simulink library "genset"  (R2014b)
settings: Solver=ode3  StartTime=0.0  StopTime=10.0  RelTol=1e-3
undefined symbols (not defined in the file): AFlowcontrol, AFn, generators, genset, i, Kappa1, ma0, magnitude, nr, pin0, swbId
libraries: goto x6, genset x3, simulink x2, switchboard x1
(part 1 of 2)
settings Model: Creator=torstebo  LastModifiedBy=torstebo

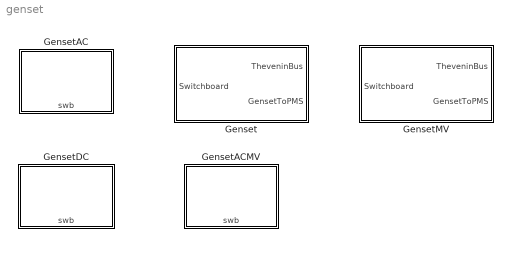
== system genset ==
  Genset : Subsystem
  GensetAC : Subsystem  Tag=GensetAC  mask{genset=generators(1), swbId=1}
      mask prompts: genset "Generator set data"; swbId "SwitchboardId"
      mask Display: image(imread('figs/generator.jpg'),'center')
  GensetACMV : Subsystem  Tag=GensetAC  mask{genset=generators(1), swbId=1}
      mask prompts: genset "Generator set data"; swbId "SwitchboardId"
      mask Display: image(imread('figs/generator.jpg'),'center')
  GensetDC : Subsystem  Tag=GensetDC  mask{genset=generators(1), swbId=1}
      mask prompts: genset "Generator set data"; swbId "SwitchboardId"
      mask Display: image(imread('figs/generator.jpg'),'center')
  GensetMV : Subsystem

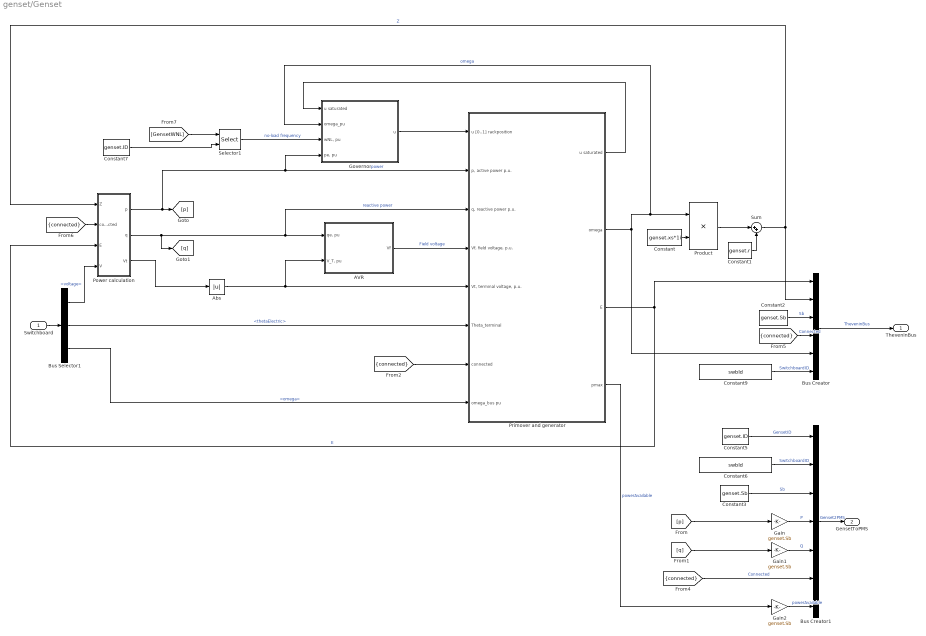
== system genset/Genset ==
  Switchboard : Inport
  AVR : Subsystem
  Abs : Abs
  Bus Creator : BusCreator  Inputs='E','Z','Sb','Connected','omega','SwitchboardID'  OutDataTypeStr=Bus: TheveninBus  NonVirtualBus=on
  Bus Creator1 : BusCreator  Inputs='GensetID','SwitchboardID','Sb','P','Q','Connected','powerAvailable'  OutDataTypeStr=Bus: Genset2PMS  NonVirtualBus=on
  Bus Selector1 : BusSelector  OutputSignals=voltage,thetaElectric,omega
  Constant : Constant  Value=genset.xs*1i
  Constant1 : Constant  Value=genset.r
  Constant2 : Constant  Value=genset.Sb
  Constant3 : Constant  Value=genset.Sb
  Constant5 : Constant  Value=genset.ID  OutDataTypeStr=Inherit: Inherit via back propagation
  Constant6 : Constant  Value=swbId  OutDataTypeStr=Inherit: Inherit via back propagation
  Constant7 : Constant  Value=genset.ID  OutDataTypeStr=Inherit: Inherit via back propagation
  Constant9 : Constant  Value=swbId  OutDataTypeStr=Inherit: Inherit via back propagation
  Gain : Gain  Gain=genset.Sb
  Gain1 : Gain  Gain=genset.Sb
  Gain2 : Gain  Gain=genset.Sb
  Governor : Subsystem
  Power calculation : MATLAB Function  TreatAsAtomicUnit=on
  Primover and generator : Subsystem
  Product : Product
  Selector1 : Selector  IndexOptions=Index vector (port)  Indices=[nr]
  Sum : Sum  Inputs=|++
  TheveninBus : Outport
  GensetToPMS : Outport  Port=2
  wires:
  Bus Selector1/2 -> Primover and generator/6(Theta_terminal)  "<thetaElectric>"
  Constant9/1 -> Bus Creator/6  "SwitchboardID"
  Switchboard/1 -> Bus Selector1/1
  Bus Selector1/3 -> Primover and generator/8(omega_bus pu)  "<omega>"
  Power calculation/3(Vt) -> Abs/1
  [connected] -> Bus Creator/4  "Connected"
  [connected] -> Bus Creator1/6  "Connected"
  [connected] -> Power calculation/2(connected)
  [connected] -> Primover and generator/7(connected)
  Gain2/1 -> Bus Creator1/7  "powerAvailable"
  Bus Selector1/1 -> Power calculation/4(V)  "<voltage>"
  Gain1/1 -> Bus Creator1/5  "Q"
  Gain/1 -> Bus Creator1/4  "P"
  Constant6/1 -> Bus Creator1/2  "SwitchboardID"
  Constant5/1 -> Bus Creator1/1  "GensetID"
  Constant3/1 -> Bus Creator1/3  "Sb"
  Selector1/1 -> Governor/3("wNL, pu")  "no-load frequency"
  AVR/1(Vf) -> Primover and generator/4("Vf, field voltage, p.u.")  "Field voltage"
  Primover and generator/1(u saturated) -> Governor/1(u saturated)
  Primover and generator/2(omega) -> Bus Creator/5, Governor/2(omega_pu), Product/1  "omega"
  Primover and generator/3(E) -> Power calculation/3(E), Bus Creator/1  "E"
  Governor/1(u) -> Primover and generator/1(u [0..1] rackposition)
  [GensetWNL] -> Selector1/1
  Power calculation/1(p) -> Primover and generator/2("p, active power p.u."), Governor/4("pe, pu"), [p]  "power"
  Power calculation/2(q) -> Primover and generator/3("q, reactive power p.u."), AVR/1("qe, pu"), [q]  "reactive power"
  Primover and generator/4(pmax) -> Gain2/1  "powerAvailable"
  Abs/1 -> Primover and generator/5("Vt, terminal voltage, p.u."), AVR/2("V_T, pu")
  Constant/1 -> Product/2
  Product/1 -> Sum/1
  Constant1/1 -> Sum/2
  Sum/1 -> Power calculation/1(Z), Bus Creator/2  "Z"
  Bus Creator/1 -> TheveninBus/1  "TheveninBus"
  Constant2/1 -> Bus Creator/3  "Sb"
  [q] -> Gain1/1
  [p] -> Gain/1
  Constant7/1 -> Selector1/2
  Bus Creator1/1 -> GensetToPMS/1  "Genset2PMS"

== system genset/GensetAC ==
  swb : Inport
  Constant4 : Constant  Value=genset.ID  OutDataTypeStr=Inherit: Inherit via back propagation
  Constant8 : Constant  Value=swbId  OutDataTypeStr=Inherit: Inherit via back propagation
  Genset : genset/Genset
      link override Primover and generator/turbo/Gain2: Gain=genset.turbo.FCdp2
      link override Primover and generator/turbo/Gain4: Gain=genset.turbo.FCdp1
  Goto Tag Visibility : GotoTagVisibility  GotoTag=connected
  Goto3 : goto/Goto  GotoTag=sprintf('Generatorset%d',genset.ID)
  Goto5 : goto/Goto  GotoTag=sprintf('GeneratorsetElectric%d',genset.ID)
  Selector : Selector  IndexOptions=Index vector (port)  Indices=[nr]
  Selector2 : Selector  IndexOptions=Index vector (port)  Indices=[nr]
  Terminator : Terminator
  tag scope: connected=scoped
  wires:
  Constant8/1 -> Selector2/2
  swb/1 -> Terminator/1
  Selector/1 -> [connected]
  [gensetsOn] -> Selector/1  "Connected"
  [switchboard] -> Selector2/1
  Constant4/1 -> Selector/2
  Selector2/1 -> Genset/1
  Genset/1 -> Goto5/1
  Genset/2 -> Goto3/1  "Genset2PMS"

== system genset/GensetACMV ==
  swb : Inport
  Constant4 : Constant  Value=genset.ID  OutDataTypeStr=Inherit: Inherit via back propagation
  Constant8 : Constant  Value=swbId  OutDataTypeStr=Inherit: Inherit via back propagation
  GensetMV : genset/GensetMV
  Goto Tag Visibility : GotoTagVisibility  GotoTag=connected
  Goto3 : goto/Goto  GotoTag=sprintf('Generatorset%d',genset.ID)
  Goto5 : goto/Goto  GotoTag=sprintf('GeneratorsetElectric%d',genset.ID)
  Selector : Selector  IndexOptions=Index vector (port)  Indices=[nr]
  Selector2 : Selector  IndexOptions=Index vector (port)  Indices=[nr]
  Terminator : Terminator
  tag scope: connected=scoped
  wires:
  Constant8/1 -> Selector2/2
  swb/1 -> Terminator/1
  Selector/1 -> [connected]
  [gensetsOn] -> Selector/1  "Connected"
  [switchboard] -> Selector2/1
  Constant4/1 -> Selector/2
  Selector2/1 -> GensetMV/1
  GensetMV/1 -> Goto5/1
  GensetMV/2 -> Goto3/1  "Genset2PMS"

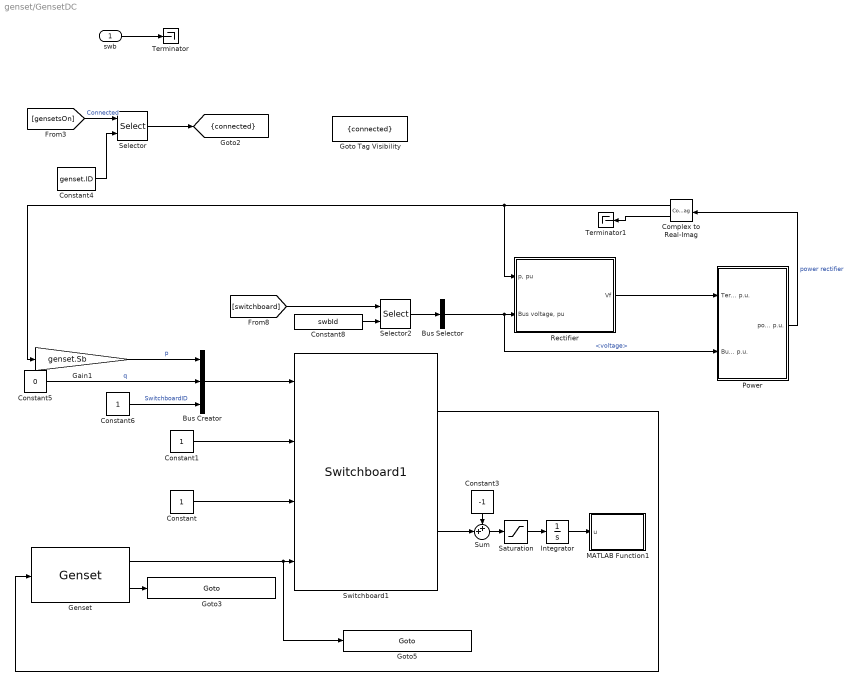
== system genset/GensetDC ==
  swb : Inport
  Bus Creator : BusCreator  Inputs=3  OutDataTypeStr=Bus: powerLoadsBus
  Bus Selector : BusSelector  OutputSignals=voltage
  Complex to Real-Imag : ComplexToRealImag
  Constant : Constant
  Constant1 : Constant
  Constant3 : Constant  Value=-1
  Constant4 : Constant  Value=genset.ID  OutDataTypeStr=Inherit: Inherit via back propagation
  Constant5 : Constant  Value=0
  Constant6 : Constant
  Constant8 : Constant  Value=swbId  OutDataTypeStr=Inherit: Inherit via back propagation
  Gain1 : Gain  Gain=genset.Sb
  Genset : genset/Genset
  Goto Tag Visibility : GotoTagVisibility  GotoTag=connected
  Goto3 : goto/Goto  GotoTag=sprintf('GeneratorsetDC%d',genset.ID)
  Goto5 : goto/Goto  GotoTag=sprintf('GeneratorsetElectricDC%d',genset.ID)
  Integrator : Integrator
  MATLAB Function1 : MATLAB Function  TreatAsAtomicUnit=on
  Power : Subsystem
  Rectifier : Subsystem
  Saturation : Saturate  UpperLimit=0  LowerLimit=-1
  Selector : Selector  IndexOptions=Index vector (port)  Indices=[nr]
  Selector2 : Selector  IndexOptions=Index vector (port)  Indices=[nr]
  Sum : Sum  Inputs=++|
  Switchboard1 : switchboard/Switchboard1
  Terminator : Terminator
  Terminator1 : Terminator
  tag scope: connected=scoped
  wires:
  Complex to Real-Imag/2 -> Terminator1/1
  Complex to Real-Imag/1 -> Gain1/1, Rectifier/1("p, pu")
  Power/1(power p.u.) -> Complex to Real-Imag/1  "power rectifier"
  Constant8/1 -> Selector2/2
  swb/1 -> Terminator/1
  Selector/1 -> [connected]
  [gensetsOn] -> Selector/1  "Connected"
  [switchboard] -> Selector2/1
  Constant4/1 -> Selector/2
  Selector2/1 -> Bus Selector/1
  Rectifier/1(Vf) -> Power/1(Terminal Voltage p.u.)
  Bus Selector/1 -> Power/2(Bus Voltage p.u.), Rectifier/2("Bus voltage, pu")  "<voltage>"
  Gain1/1 -> Bus Creator/1  "p"
  Bus Creator/1 -> Switchboard1/1
  Constant3/1 -> Sum/1
  Constant5/1 -> Bus Creator/2  "q"
  Integrator/1 -> MATLAB Function1/1(u)
  Constant/1 -> Switchboard1/3
  Sum/1 -> Saturation/1
  Saturation/1 -> Integrator/1
  Switchboard1/1 -> Genset/1
  Constant6/1 -> Bus Creator/3  "SwitchboardID"
  Switchboard1/2 -> Sum/2
  Constant1/1 -> Switchboard1/2
  Genset/1 -> Goto5/1, Switchboard1/4
  Genset/2 -> Goto3/1

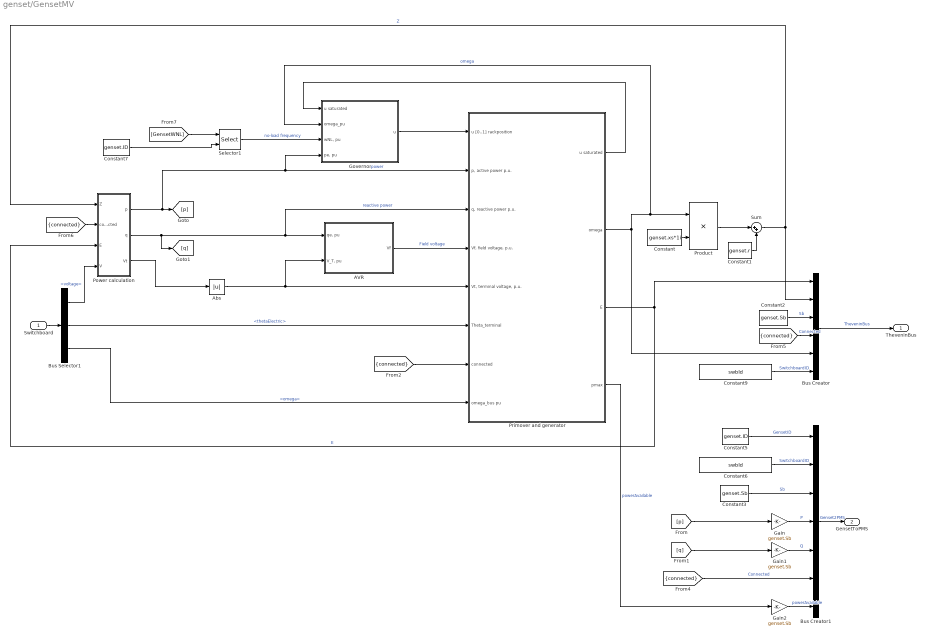
== system genset/GensetMV ==
  Switchboard : Inport
  AVR : Subsystem
  Abs : Abs
  Bus Creator : BusCreator  Inputs='E','Z','Sb','Connected','omega','SwitchboardID'  OutDataTypeStr=Bus: TheveninBus  NonVirtualBus=on
  Bus Creator1 : BusCreator  Inputs='GensetID','SwitchboardID','Sb','P','Q','Connected','powerAvailable'  OutDataTypeStr=Bus: Genset2PMS  NonVirtualBus=on
  Bus Selector1 : BusSelector  OutputSignals=voltage,thetaElectric,omega
  Constant : Constant  Value=genset.xs*1i
  Constant1 : Constant  Value=genset.r
  Constant2 : Constant  Value=genset.Sb
  Constant3 : Constant  Value=genset.Sb
  Constant5 : Constant  Value=genset.ID  OutDataTypeStr=Inherit: Inherit via back propagation
  Constant6 : Constant  Value=swbId  OutDataTypeStr=Inherit: Inherit via back propagation
  Constant7 : Constant  Value=genset.ID  OutDataTypeStr=Inherit: Inherit via back propagation
  Constant9 : Constant  Value=swbId  OutDataTypeStr=Inherit: Inherit via back propagation
  Gain : Gain  Gain=genset.Sb
  Gain1 : Gain  Gain=genset.Sb
  Gain2 : Gain  Gain=genset.Sb
  Governor : Subsystem
  Power calculation : MATLAB Function  TreatAsAtomicUnit=on
  Primover and generator : Subsystem
  Product : Product
  Selector1 : Selector  IndexOptions=Index vector (port)  Indices=[nr]
  Sum : Sum  Inputs=|++
  TheveninBus : Outport
  GensetToPMS : Outport  Port=2
  wires:
  Bus Selector1/2 -> Primover and generator/6(Theta_terminal)  "<thetaElectric>"
  Constant9/1 -> Bus Creator/6  "SwitchboardID"
  Switchboard/1 -> Bus Selector1/1
  Bus Selector1/3 -> Primover and generator/8(omega_bus pu)  "<omega>"
  Power calculation/3(Vt) -> Abs/1
  [connected] -> Bus Creator/4  "Connected"
  [connected] -> Bus Creator1/6  "Connected"
  [connected] -> Power calculation/2(connected)
  [connected] -> Primover and generator/7(connected)
  Gain2/1 -> Bus Creator1/7  "powerAvailable"
  Bus Selector1/1 -> Power calculation/4(V)  "<voltage>"
  Gain1/1 -> Bus Creator1/5  "Q"
  Gain/1 -> Bus Creator1/4  "P"
  Constant6/1 -> Bus Creator1/2  "SwitchboardID"
  Constant5/1 -> Bus Creator1/1  "GensetID"
  Constant3/1 -> Bus Creator1/3  "Sb"
  Selector1/1 -> Governor/3("wNL, pu")  "no-load frequency"
  AVR/1(Vf) -> Primover and generator/4("Vf, field voltage, p.u.")  "Field voltage"
  Primover and generator/1(u saturated) -> Governor/1(u saturated)
  Primover and generator/2(omega) -> Bus Creator/5, Governor/2(omega_pu), Product/1  "omega"
  Primover and generator/3(E) -> Power calculation/3(E), Bus Creator/1  "E"
  Governor/1(u) -> Primover and generator/1(u [0..1] rackposition)
  [GensetWNL] -> Selector1/1
  Power calculation/1(p) -> Primover and generator/2("p, active power p.u."), Governor/4("pe, pu"), [p]  "power"
  Power calculation/2(q) -> Primover and generator/3("q, reactive power p.u."), AVR/1("qe, pu"), [q]  "reactive power"
  Primover and generator/4(pmax) -> Gain2/1  "powerAvailable"
  Abs/1 -> Primover and generator/5("Vt, terminal voltage, p.u."), AVR/2("V_T, pu")
  Constant/1 -> Product/2
  Product/1 -> Sum/1
  Constant1/1 -> Sum/2
  Sum/1 -> Power calculation/1(Z), Bus Creator/2  "Z"
  Bus Creator/1 -> TheveninBus/1  "TheveninBus"
  Constant2/1 -> Bus Creator/3  "Sb"
  [q] -> Gain1/1
  [p] -> Gain/1
  Constant7/1 -> Selector1/2
  Bus Creator1/1 -> GensetToPMS/1  "Genset2PMS"

== system genset/Genset/AVR ==
  "qe, pu" : Inport
  "V_T, pu" : Inport  Port=2
  Constant : Constant
  Constant7 : Constant  Value=genset.ID  OutDataTypeStr=Inherit: Inherit via back propagation
  Gain : Gain  Gain=genset.avr.droop
  Low pass filter : Subsystem
  PI controller : Subsystem
  Product : Product  RndMeth=Zero
  Selector1 : Selector  IndexOptions=Index vector (port)  Indices=[nr]
  Sum1 : Sum  Inputs=|+-
  Sum3 : Sum  Inputs=|+-
  Vf : Outport
  wires:
  Selector1/1 -> Product/1  "no-load frequency"
  [GensetVNL] -> Selector1/1
  Constant7/1 -> Selector1/2
  PI controller/1(vf) -> Low pass filter/1(V)
  Sum1/1 -> PI controller/1(e)
  "qe, pu"/1 -> Gain/1
  "V_T, pu"/1 -> Sum1/2
  Constant/1 -> Sum3/1
  Gain/1 -> Sum3/2
  Sum3/1 -> Product/2
  Product/1 -> Sum1/1
  Low pass filter/1(Vold) -> Vf/1

== system genset/Genset/Governor ==
  u saturated : Inport
  omega_pu : Inport  Port=2
  "wNL, pu" : Inport  Port=3
  "pe, pu" : Inport  Port=4
  Constant : Constant
  Gain : Gain  Gain=genset.governor.droop
  PID controller : Subsystem
  Product : Product  RndMeth=Zero
  Sum : Sum  Inputs=|+-
  Sum1 : Sum  Inputs=|+-
  u : Outport
  wires:
  PID controller/1(u) -> u/1  "u"
  Gain/1 -> Sum1/2
  Sum/1 -> PID controller/1(e)
  Product/1 -> Sum/1
  "wNL, pu"/1 -> Product/1
  Constant/1 -> Sum1/1
  Sum1/1 -> Product/2
  u saturated/1 -> PID controller/3(u saturated)
  "pe, pu"/1 -> Gain/1
  omega_pu/1 -> Sum/2, PID controller/2(omega_pu)

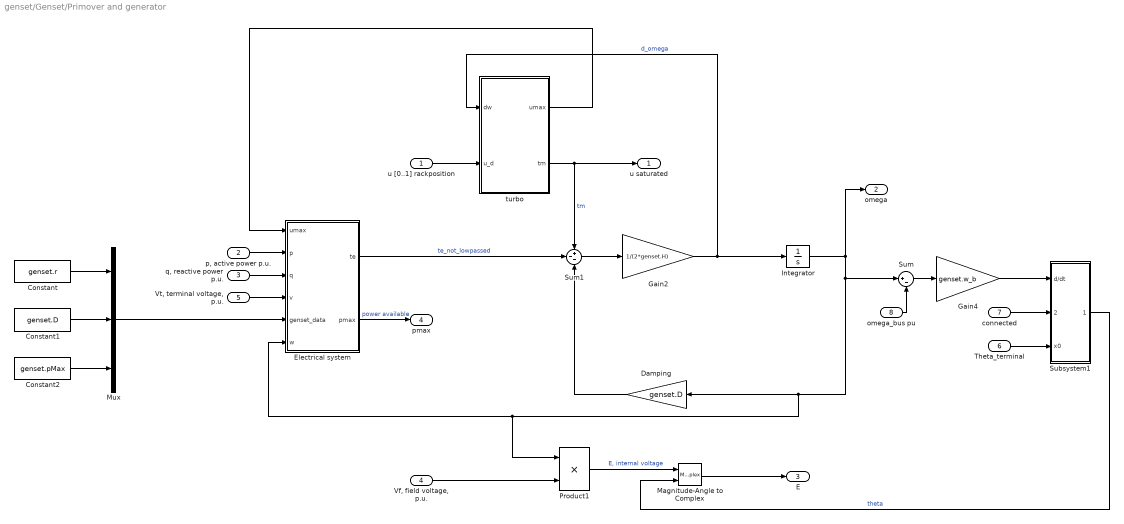
== system genset/Genset/Primover and generator ==
  u [0..1] rackposition : Inport
  "p, active power p.u." : Inport  Port=2
  "q, reactive power p.u." : Inport  Port=3
  "Vf, field voltage, p.u." : Inport  Port=4
  "Vt, terminal voltage, p.u." : Inport  Port=5
  Theta_terminal : Inport  Port=6
  connected : Inport  Port=7
  omega_bus pu : Inport  Port=8
  Constant : Constant  Value=genset.r
  Constant1 : Constant  Value=genset.D
  Constant2 : Constant  Value=genset.pMax
  Damping : Gain  Gain=genset.D
  Electrical system : MATLAB Function  TreatAsAtomicUnit=on
  Gain2 : Gain  Gain=1/(2*genset.H)
  Gain4 : Gain  Gain=genset.w_b
  Integrator : Integrator  InitialCondition=genset.omega0
  Magnitude-Angle to Complex : MagnitudeAngleToComplex
  Mux : Mux  Inputs=3
  Product1 : Product  Inputs=**  RndMeth=Zero
  Subsystem1 : Subsystem
  Sum : Sum  Inputs=|+-
  Sum1 : Sum  Inputs=+--
  turbo : Subsystem
  u saturated : Outport
  omega : Outport  Port=2
  E : Outport  Port=3
  pmax : Outport  Port=4
  wires:
  omega_bus pu/1 -> Sum/2
  Sum/1 -> Gain4/1
  u [0..1] rackposition/1 -> turbo/2(u_d)
  turbo/2(tm) -> u saturated/1, Sum1/1  "tm"
  Product1/1 -> Magnitude-Angle to Complex/1  "E, internal voltage"
  Subsystem1/1(Out1) -> Magnitude-Angle to Complex/2  "theta"
  Gain4/1 -> Subsystem1/1(d/dt)
  Sum1/1 -> Gain2/1
  Gain2/1 -> turbo/1(dw), Integrator/1  "d_omega"
  "Vf, field voltage, p.u."/1 -> Product1/2
  "p, active power p.u."/1 -> Electrical system/2(p)
  Electrical system/1(te) -> Sum1/2  "te_not_lowpassed"
  "Vt, terminal voltage, p.u."/1 -> Electrical system/4(v)
  "q, reactive power p.u."/1 -> Electrical system/3(q)
  Damping/1 -> Sum1/3
  connected/1 -> Subsystem1/2(reset)
  Integrator/1 -> Sum/1, Damping/1, Product1/1, Electrical system/6(w), omega/1
  Theta_terminal/1 -> Subsystem1/3(x0)
  turbo/1(umax) -> Electrical system/1(umax)
  Electrical system/2(pmax) -> pmax/1  "power available"
  Magnitude-Angle to Complex/1 -> E/1
  Constant/1 -> Mux/1
  Constant1/1 -> Mux/2
  Constant2/1 -> Mux/3
  Mux/1 -> Electrical system/5(genset_data)

== system genset/GensetDC/Power ==
  Terminal Voltage p.u. : Inport
  Bus Voltage p.u. : Inport  Port=2
  Gain : Gain  Gain=1/genset.rectifier.r
  Product : Product
  Sum1 : Sum  Inputs=+|-
  power p.u. : Outport
  wires:
  Gain/1 -> Product/2  "current"
  Sum1/1 -> Gain/1
  Bus Voltage p.u./1 -> Sum1/2
  Terminal Voltage p.u./1 -> Product/1, Sum1/1
  Product/1 -> power p.u./1

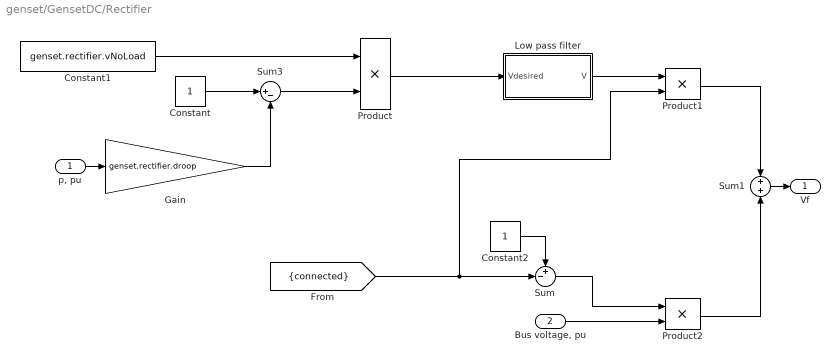
== system genset/GensetDC/Rectifier ==
  "p, pu" : Inport
  "Bus voltage, pu" : Inport  Port=2
  Constant : Constant
  Constant1 : Constant  Value=genset.rectifier.vNoLoad
  Constant2 : Constant
  Gain : Gain  Gain=genset.rectifier.droop
  Low pass filter : Subsystem
  Product : Product  RndMeth=Zero
  Product1 : Product
  Product2 : Product
  Sum : Sum  Inputs=+-|
  Sum1 : Sum
  Sum3 : Sum  Inputs=|+-
  Vf : Outport
  wires:
  Product/1 -> Low pass filter/1(Vdesired)
  "p, pu"/1 -> Gain/1
  Constant1/1 -> Product/1
  Constant/1 -> Sum3/1
  Gain/1 -> Sum3/2
  Sum3/1 -> Product/2
  Low pass filter/1(V) -> Product1/1
  "Bus voltage, pu"/1 -> Product2/2
  [connected] -> Product1/2, Sum/2
  Constant2/1 -> Sum/1
  Sum/1 -> Product2/1
  Product2/1 -> Sum1/2
  Product1/1 -> Sum1/1
  Sum1/1 -> Vf/1

== system genset/GensetMV/AVR ==
  "qe, pu" : Inport
  "V_T, pu" : Inport  Port=2
  Constant : Constant
  Constant7 : Constant  Value=genset.ID  OutDataTypeStr=Inherit: Inherit via back propagation
  Gain : Gain  Gain=genset.avr.droop
  Low pass filter : Subsystem
  PI controller : Subsystem
  Product : Product  RndMeth=Zero
  Selector1 : Selector  IndexOptions=Index vector (port)  Indices=[nr]
  Sum1 : Sum  Inputs=|+-
  Sum3 : Sum  Inputs=|+-
  Vf : Outport
  wires:
  Selector1/1 -> Product/1  "no-load frequency"
  [GensetVNL] -> Selector1/1
  Constant7/1 -> Selector1/2
  PI controller/1(vf) -> Low pass filter/1(V)
  Sum1/1 -> PI controller/1(e)
  "qe, pu"/1 -> Gain/1
  "V_T, pu"/1 -> Sum1/2
  Constant/1 -> Sum3/1
  Gain/1 -> Sum3/2
  Sum3/1 -> Product/2
  Product/1 -> Sum1/1
  Low pass filter/1(Vold) -> Vf/1

== system genset/GensetMV/Governor ==
  u saturated : Inport
  omega_pu : Inport  Port=2
  "wNL, pu" : Inport  Port=3
  "pe, pu" : Inport  Port=4
  Constant : Constant
  Gain : Gain  Gain=genset.governor.droop
  PID controller : Subsystem
  Product : Product  RndMeth=Zero
  Sum : Sum  Inputs=|+-
  Sum1 : Sum  Inputs=|+-
  u : Outport
  wires:
  PID controller/1(u) -> u/1  "u"
  Gain/1 -> Sum1/2
  Sum/1 -> PID controller/1(e)
  Product/1 -> Sum/1
  "wNL, pu"/1 -> Product/1
  Constant/1 -> Sum1/1
  Sum1/1 -> Product/2
  u saturated/1 -> PID controller/3(u saturated)
  "pe, pu"/1 -> Gain/1
  omega_pu/1 -> Sum/2, PID controller/2(omega_pu)

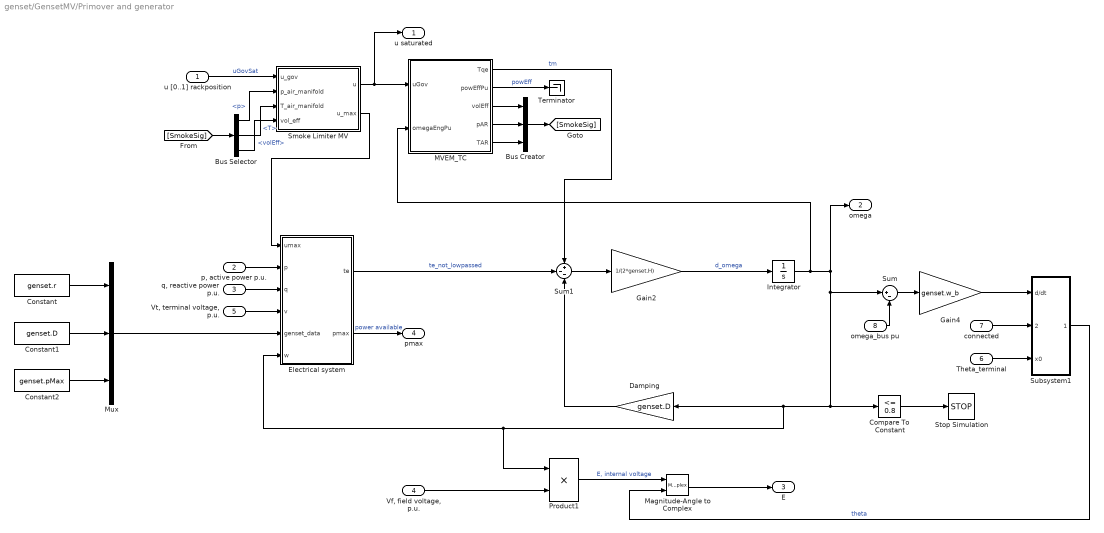
== system genset/GensetMV/Primover and generator ==
  u [0..1] rackposition : Inport
  "p, active power p.u." : Inport  Port=2
  "q, reactive power p.u." : Inport  Port=3
  "Vf, field voltage, p.u." : Inport  Port=4
  "Vt, terminal voltage, p.u." : Inport  Port=5
  Theta_terminal : Inport  Port=6
  connected : Inport  Port=7
  omega_bus pu : Inport  Port=8
  Bus Creator : BusCreator  Inputs=3
  Bus Selector : BusSelector  OutputSignals=p,T,volEff
  Compare To Constant : simulink/Logic and Bit Operations/Compare To Constant  relop=<=  const=0.8  OutDataTypeStr=boolean
  Constant : Constant  Value=genset.r
  Constant1 : Constant  Value=genset.D
  Constant2 : Constant  Value=genset.pMax
  Damping : Gain  Gain=genset.D
  Electrical system : MATLAB Function  TreatAsAtomicUnit=on
  Gain2 : Gain  Gain=1/(2*genset.H)
  Gain4 : Gain  Gain=genset.w_b
  Integrator : Integrator  InitialCondition=genset.omega0
  MVEM_TC : Subsystem  mask{genset=genset}
      mask prompts: genset "Genset parameters"
  Magnitude-Angle to Complex : MagnitudeAngleToComplex
  Mux : Mux  Inputs=3
  Product1 : Product  Inputs=**  RndMeth=Zero
  Smoke Limiter MV : Subsystem  mask{fs=genset.eng.fs, Vd=genset.eng.vD, F_max=genset.eng.fMax, m_f_cyc_max=genset.eng.mFCycMax, p0AR=genset.eng.p0AR, T0AR=genset.eng.T0AR, vol_eff_coeff=genset.eng.volEff}
      mask prompts: fs "Stoichiometric fuel-air ratio"; Vd "Displacement volume (m3)"; F_max "Maximum fuel-air equivalent ratio"; m_f_cyc_max "Maximum fuel injection @ rated power (kg)"; p0AR "Initial pressure at manifold"; T0AR "Initial temperature at manifold"; vol_eff_coeff "Volumetric efficiency coefficient"
  Stop Simulation : Stop
  Subsystem1 : Subsystem
  Sum : Sum  Inputs=|+-
  Sum1 : Sum  Inputs=+--
  Terminator : Terminator
  u saturated : Outport
  omega : Outport  Port=2
  E : Outport  Port=3
  pmax : Outport  Port=4
  wires:
  Compare To Constant/1 -> Stop Simulation/1
  Smoke Limiter MV/2(u_max) -> Electrical system/1(umax)
  Bus Selector/3 -> Smoke Limiter MV/4(vol_eff)  "<volEff>"
  Bus Selector/1 -> Smoke Limiter MV/2(p_air_manifold)  "<p>"
  Bus Selector/2 -> Smoke Limiter MV/3(T_air_manifold)  "<T>"
  [SmokeSig] -> Bus Selector/1
  u [0..1] rackposition/1 -> Smoke Limiter MV/1(u_gov)  "uGovSat"
  Smoke Limiter MV/1(u) -> MVEM_TC/1(uGov), u saturated/1
  MVEM_TC/5(TAR) -> Bus Creator/3
  MVEM_TC/3(volEff) -> Bus Creator/1
  Bus Creator/1 -> [SmokeSig]
  MVEM_TC/2(powEffPu) -> Terminator/1  "powEff"
  MVEM_TC/4(pAR) -> Bus Creator/2
  omega_bus pu/1 -> Sum/2
  Sum/1 -> Gain4/1
  MVEM_TC/1(Tqe) -> Sum1/1  "tm"
  Product1/1 -> Magnitude-Angle to Complex/1  "E, internal voltage"
  Subsystem1/1(Out1) -> Magnitude-Angle to Complex/2  "theta"
  Gain4/1 -> Subsystem1/1(d/dt)
  Sum1/1 -> Gain2/1
  Gain2/1 -> Integrator/1  "d_omega"
  "Vf, field voltage, p.u."/1 -> Product1/2
  "p, active power p.u."/1 -> Electrical system/2(p)
  Electrical system/1(te) -> Sum1/2  "te_not_lowpassed"
  "Vt, terminal voltage, p.u."/1 -> Electrical system/4(v)
  "q, reactive power p.u."/1 -> Electrical system/3(q)
  Damping/1 -> Sum1/3
  connected/1 -> Subsystem1/2(reset)
  Integrator/1 -> Sum/1, Damping/1, Product1/1, Electrical system/6(w), Compare To Constant/1, omega/1, MVEM_TC/2(omegaEngPu)
  Theta_terminal/1 -> Subsystem1/3(x0)
  Electrical system/2(pmax) -> pmax/1  "power available"
  Magnitude-Angle to Complex/1 -> E/1
  Constant/1 -> Mux/1
  Constant1/1 -> Mux/2
  Constant2/1 -> Mux/3
  Mux/1 -> Electrical system/5(genset_data)

== system genset/Genset/AVR/Low pass filter ==
  V : Inport
  Gain : Gain  Gain=1/genset.avr.T
  Integrator : Integrator  InitialCondition=genset.avr.v0
  Sum : Sum  Inputs=|+-
  Vold : Outport
  wires:
  Integrator/1 -> Vold/1, Sum/2
  V/1 -> Sum/1
  Sum/1 -> Gain/1
  Gain/1 -> Integrator/1

== system genset/Genset/AVR/PI controller ==
  e : Inport
  Gain : Gain  Gain=genset.avr.ki
  Gain1 : Gain  Gain=genset.avr.kp
  Integrator : Integrator  DisableCoverage=on  InitialCondition=genset.avr.v0
  Saturation : Saturate  UpperLimit=genset.avr.maxFieldVoltage  LowerLimit=genset.avr.minFieldVoltage  LinearizeAsGain=off  OutMin=genset.avr.minFieldVoltage  OutMax=genset.avr.maxFieldVoltage  OutDataTypeStr=Inherit: Inherit via back propagation
  Sum : Sum  Inputs=+|+
  vf : Outport
  wires:
  Saturation/1 -> vf/1
  Sum/1 -> Saturation/1
  e/1 -> Gain/1, Gain1/1
  Integrator/1 -> Sum/2
  Gain1/1 -> Sum/1
  Gain/1 -> Integrator/1

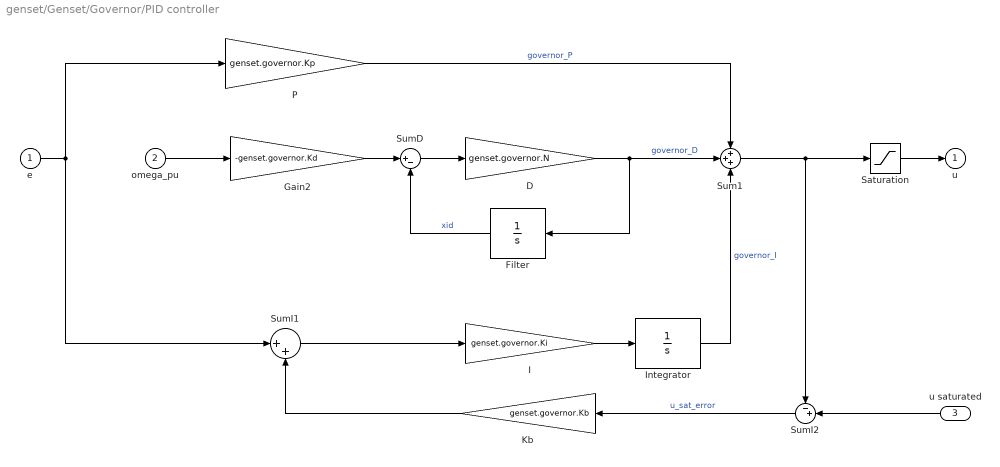
== system genset/Genset/Governor/PID controller ==
  e : Inport  PortDimensions=1
  omega_pu : Inport  Port=2  PortDimensions=1
  u saturated : Inport  Port=3  PortDimensions=1
  D : Gain  DisableCoverage=on  Gain=genset.governor.N
  Filter : Integrator  DisableCoverage=on  InitialCondition=-genset.omega0*genset.governor.Kd
  Gain2 : Gain  Gain=-genset.governor.Kd
  I : Gain  Gain=genset.governor.Ki
  Integrator : Integrator  DisableCoverage=on  InitialCondition=genset.u0
  Kb : Gain  DisableCoverage=on  Gain=genset.governor.Kb  ParamDataTypeStr=Inherit: Inherit from 'Gain'
  P : Gain  Gain=genset.governor.Kp
  Saturation : Saturate  UpperLimit=genset.uMax  LowerLimit=genset.uMin  LinearizeAsGain=off  OutMin=genset.uMin  OutMax=genset.uMax  OutDataTypeStr=Inherit: Inherit via back propagation
  Sum1 : Sum  Inputs=+++
  SumD : Sum  DisableCoverage=on  Inputs=|+-
  SumI1 : Sum  DisableCoverage=on  Inputs=|++
  SumI2 : Sum  DisableCoverage=on  Inputs=-+|
  u : Outport  PortDimensions=1  InitialOutput=0
  wires:
  Integrator/1 -> Sum1/3  "governor_I"
  D/1 -> Sum1/2, Filter/1  "governor_D"
  omega_pu/1 -> Gain2/1
  e/1 -> P/1, SumI1/1
  P/1 -> Sum1/1  "governor_P"
  Saturation/1 -> u/1
  Filter/1 -> SumD/2  "xid"
  SumD/1 -> D/1
  Gain2/1 -> SumD/1
  Sum1/1 -> Saturation/1, SumI2/1
  SumI2/1 -> Kb/1  "u_sat_error"
  Kb/1 -> SumI1/2
  u saturated/1 -> SumI2/2
  SumI1/1 -> I/1
  I/1 -> Integrator/1

== system genset/Genset/Primover and generator/Subsystem1 ==
  d/dt : Inport
  reset : Inport  Port=2
  x0 : Inport  Port=3
  Gain : Gain  Gain=1000
  Integrator : Integrator  InitialCondition=genset.theta0
  MATLAB Function : MATLAB Function  TreatAsAtomicUnit=on
  Sum : Sum  Inputs=-|+
  Switch : Switch  Threshold=1
  Out1 : Outport
  wires:
  Integrator/1 -> Out1/1, Sum/1
  reset/1 -> Switch/2
  x0/1 -> Sum/2
  Sum/1 -> MATLAB Function/1(u)
  Gain/1 -> Switch/3
  MATLAB Function/1(y) -> Gain/1
  d/dt/1 -> Switch/1
  Switch/1 -> Integrator/1

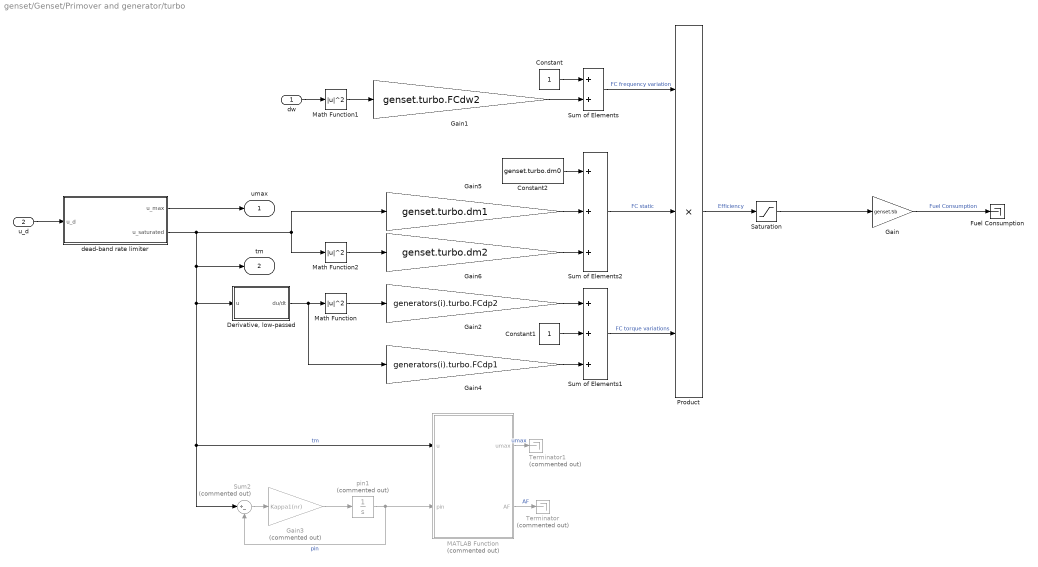
== system genset/Genset/Primover and generator/turbo ==
  dw : Inport
  u_d : Inport  Port=2
  Constant : Constant
  Constant1 : Constant
  Constant2 : Constant  Value=genset.turbo.dm0
  "Derivative, low-passed" : Subsystem
      settings: MinAlgLoopOccurrences=on
  Fuel Consumption : Terminator
  Gain : Gain  Gain=genset.Sb
  Gain1 : Gain  Gain=genset.turbo.FCdw2
  Gain2 : Gain  Gain=generators(i).turbo.FCdp2
  Gain3 : Gain  Commented=on  Gain=Kappa1(nr)
  Gain4 : Gain  Gain=generators(i).turbo.FCdp1
  Gain5 : Gain  Gain=genset.turbo.dm1
  Gain6 : Gain  Gain=genset.turbo.dm2
  MATLAB Function : MATLAB Function  Commented=on  TreatAsAtomicUnit=on
  Math Function : Math  Operator=magnitude^2  SaturateOnIntegerOverflow=on
  Math Function1 : Math  Operator=magnitude^2  SaturateOnIntegerOverflow=on
  Math Function2 : Math  Operator=magnitude^2  SaturateOnIntegerOverflow=on
  Product : Product  Inputs=3  RndMeth=Zero
  Saturation : Saturate  UpperLimit=genset.turbo.FCmax  LowerLimit=0
  Sum of Elements : Sum
  Sum of Elements1 : Sum  Inputs=+++
  Sum of Elements2 : Sum  Inputs=+++
  Sum2 : Sum  Commented=on  Inputs=|+-
  Terminator : Terminator  Commented=on
  Terminator1 : Terminator  Commented=on
  dead-band rate limiter : Subsystem  mask(Rate limiter for diesel engines){umax=genset.uMax, umin=genset.uMin}
      mask prompts: umax "Static maximum torque"; umin "Static minimum torque"
      mask help:
      | Allows the input to change within a delta limit, however if the input
      | changes more than this range will the input be saturated by a rate limiter.
  pin1 : Integrator  Commented=on  InitialCondition=pin0(nr)
  umax : Outport
  tm : Outport  Port=2
  wires:
  Gain/1 -> Fuel Consumption/1  "Fuel Consumption"
  Saturation/1 -> Gain/1
  Product/1 -> Saturation/1  "Efficiency"
  Sum of Elements/1 -> Product/1  "FC frequency variation"
  Sum of Elements2/1 -> Product/2  "FC static"
  Sum of Elements1/1 -> Product/3  "FC torque variations"
  Math Function2/1 -> Gain6/1
  Constant2/1 -> Sum of Elements2/1
  Gain5/1 -> Sum of Elements2/2
  Gain6/1 -> Sum of Elements2/3
  Constant1/1 -> Sum of Elements1/2
  Gain4/1 -> Sum of Elements1/3
  Gain2/1 -> Sum of Elements1/1
  Constant/1 -> Sum of Elements/1
  Gain1/1 -> Sum of Elements/2
  Math Function/1 -> Gain2/1
  Math Function1/1 -> Gain1/1
  "Derivative, low-passed"/1(du/dt) -> Math Function/1, Gain4/1
  pin1/1 -> MATLAB Function/2(pin), Sum2/2  "pin"
  Sum2/1 -> Gain3/1
  Gain3/1 -> pin1/1
  dead-band rate limiter/2(u_saturated) -> tm/1, Sum2/1, MATLAB Function/1(u), "Derivative, low-passed"/1(u), Gain5/1, Math Function2/1  "tm"
  u_d/1 -> dead-band rate limiter/1(u_d)
  MATLAB Function/2(AF) -> Terminator/1  "AF"
  dw/1 -> Math Function1/1
  MATLAB Function/1(umax) -> Terminator1/1  "umax"
  dead-band rate limiter/1(u_max) -> umax/1

== system genset/GensetDC/Rectifier/Low pass filter ==
  Vdesired : Inport
  Gain : Gain  Gain=1/genset.rectifier.t
  Integrator : Integrator  InitialCondition=genset.rectifier.v0
  Sum : Sum  Inputs=|+-
  V : Outport
  wires:
  Integrator/1 -> V/1, Sum/2
  Vdesired/1 -> Sum/1
  Sum/1 -> Gain/1
  Gain/1 -> Integrator/1

== system genset/GensetMV/AVR/Low pass filter ==
  V : Inport
  Gain : Gain  Gain=1/genset.avr.T
  Integrator : Integrator  InitialCondition=genset.avr.v0
  Sum : Sum  Inputs=|+-
  Vold : Outport
  wires:
  Integrator/1 -> Vold/1, Sum/2
  V/1 -> Sum/1
  Sum/1 -> Gain/1
  Gain/1 -> Integrator/1

== system genset/GensetMV/AVR/PI controller ==
  e : Inport
  Gain : Gain  Gain=genset.avr.ki
  Gain1 : Gain  Gain=genset.avr.kp
  Integrator : Integrator  DisableCoverage=on  InitialCondition=genset.avr.v0
  Saturation : Saturate  UpperLimit=genset.avr.maxFieldVoltage  LowerLimit=genset.avr.minFieldVoltage  LinearizeAsGain=off  OutMin=genset.avr.minFieldVoltage  OutMax=genset.avr.maxFieldVoltage  OutDataTypeStr=Inherit: Inherit via back propagation
  Sum : Sum  Inputs=+|+
  vf : Outport
  wires:
  Saturation/1 -> vf/1
  Sum/1 -> Saturation/1
  e/1 -> Gain/1, Gain1/1
  Integrator/1 -> Sum/2
  Gain1/1 -> Sum/1
  Gain/1 -> Integrator/1

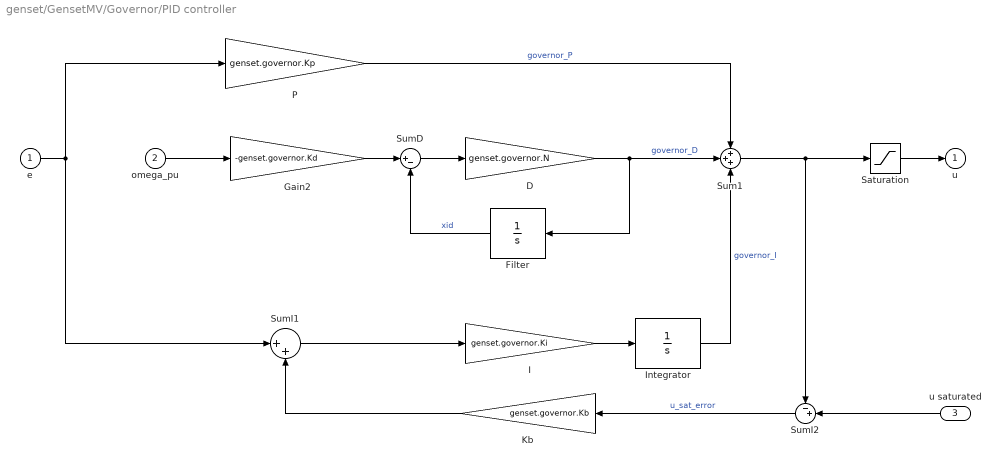
== system genset/GensetMV/Governor/PID controller ==
  e : Inport  PortDimensions=1
  omega_pu : Inport  Port=2  PortDimensions=1
  u saturated : Inport  Port=3  PortDimensions=1
  D : Gain  DisableCoverage=on  Gain=genset.governor.N
  Filter : Integrator  DisableCoverage=on  InitialCondition=-genset.omega0*genset.governor.Kd
  Gain2 : Gain  Gain=-genset.governor.Kd
  I : Gain  Gain=genset.governor.Ki
  Integrator : Integrator  DisableCoverage=on  InitialCondition=genset.u0
  Kb : Gain  DisableCoverage=on  Gain=genset.governor.Kb  ParamDataTypeStr=Inherit: Inherit from 'Gain'
  P : Gain  Gain=genset.governor.Kp
  Saturation : Saturate  UpperLimit=genset.uMax  LowerLimit=genset.uMin  LinearizeAsGain=off  OutMin=genset.uMin  OutMax=genset.uMax  OutDataTypeStr=Inherit: Inherit via back propagation
  Sum1 : Sum  Inputs=+++
  SumD : Sum  DisableCoverage=on  Inputs=|+-
  SumI1 : Sum  DisableCoverage=on  Inputs=|++
  SumI2 : Sum  DisableCoverage=on  Inputs=-+|
  u : Outport  PortDimensions=1  InitialOutput=0
  wires:
  Integrator/1 -> Sum1/3  "governor_I"
  D/1 -> Sum1/2, Filter/1  "governor_D"
  omega_pu/1 -> Gain2/1
  e/1 -> P/1, SumI1/1
  P/1 -> Sum1/1  "governor_P"
  Saturation/1 -> u/1
  Filter/1 -> SumD/2  "xid"
  SumD/1 -> D/1
  Gain2/1 -> SumD/1
  Sum1/1 -> Saturation/1, SumI2/1
  SumI2/1 -> Kb/1  "u_sat_error"
  Kb/1 -> SumI1/2
  u saturated/1 -> SumI2/2
  SumI1/1 -> I/1
  I/1 -> Integrator/1

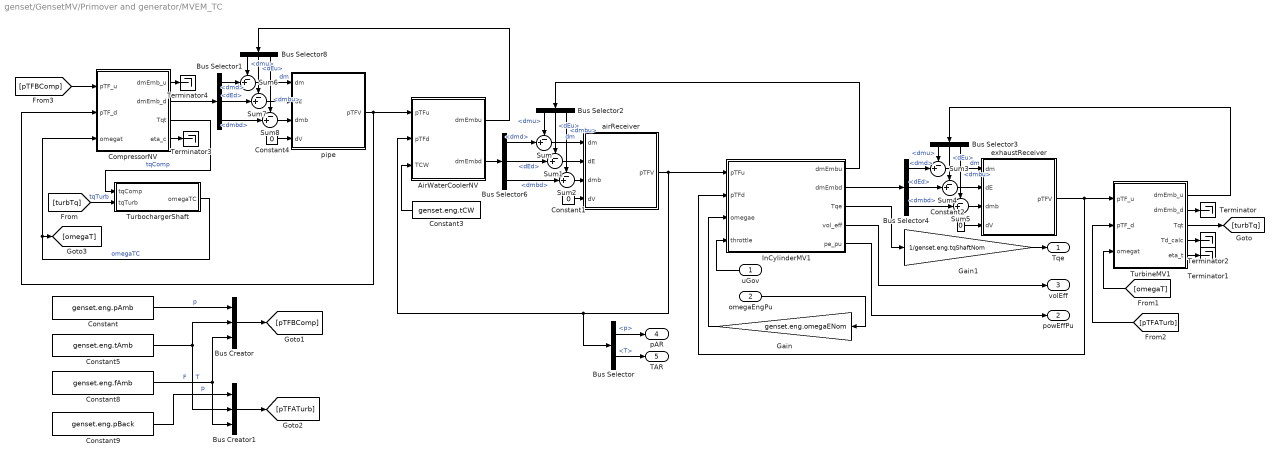
== system genset/GensetMV/Primover and generator/MVEM_TC ==
  uGov : Inport
  omegaEngPu : Inport  Port=2
  AirWaterCoolerNV : Subsystem  mask{fs=genset.eng.fs, Cd=genset.eng.cdCool, A_air_path=genset.eng.aAirPath, dm_cw=genset.eng.dmCW, coeff_T_cw_K=genset.eng.coeffKTCW, Cp_cw=genset.eng.cpCW, D_cw_pipe=genset.eng.dPipeCW}
      mask prompts: fs "Stoichiometric fuel-air ratio"; Cd "Discharge coefficient (0.8)"; A_air_path "Effective sectional area of air path (m2)"; dm_cw "Coolant flow rate (kg/s)"; coeff_T_cw_K "Coefficient for effective heat transfer area w.r.t. coolant temperature (2x1)"; Cp_cw "Specific heat capacity of coolant"; D_cw_pipe "Pipe diameter of the cooling water pipe in the cooler (m)"
      mask TypeOptions fs: S-Function/fs
      mask TypeOptions Cd: S-Function/Cd
      mask TypeOptions A_air_path: S-Function/A_air_path
      mask TypeOptions dm_cw: S-Function/dm_cw
      mask TypeOptions coeff_T_cw_K: S-Function/coeff_T_cw_K
      mask TypeOptions Cp_cw: S-Function/Cp_cw
      mask TypeOptions D_cw_pipe: S-Function/D_cw_pipe
      mask Display: image(imread('figs/cooler.png'),'center')
  Bus Creator : BusCreator  Inputs=3
  Bus Creator1 : BusCreator  Inputs=3
  Bus Selector : BusSelector  OutputSignals=p,T
  Bus Selector1 : BusSelector  OutputSignals=dmd,dEd,dmbd
  Bus Selector2 : BusSelector  OutputSignals=dmu,dEu,dmbu
  Bus Selector3 : BusSelector  OutputSignals=dmu,dEu,dmbu
  Bus Selector4 : BusSelector  OutputSignals=dmd,dEd,dmbd
  Bus Selector6 : BusSelector  OutputSignals=dmd,dEd,dmbd
  Bus Selector8 : BusSelector  OutputSignals=dmu,dEu,dmbu
  CompressorNV : Subsystem  mask{fs=genset.eng.fs, comp_flow_map=genset.eng.compFlowMap, comp_eff_map=genset.eng.compEffMap, pr_rep=genset.eng.prRep, n288_rep=genset.eng.n288Rep, npr=genset.eng.npr, nsp=genset.eng.nsp}
      mask prompts: fs "Fuel-air equivalent ratio"; comp_flow_map "Compressor map for corrected flow"; comp_eff_map "Compressor map for efficiency"; pr_rep "Pressure ratio array for look-up in compressor map"; n288_rep "Corrected speed array for look-up in compressor map"; npr "Length of pressure ratio array for look-up in compressor map"; nsp "Length of corrected speed array for look-up in compressor map"
      mask Display: image(imread('figs/Compressor.png'),'center')
  Constant : Constant  Value=genset.eng.pAmb
  Constant1 : Constant  Value=0
  Constant2 : Constant  Value=0
  Constant3 : Constant  Value=genset.eng.tCW
  Constant4 : Constant  Value=0
  Constant5 : Constant  Value=genset.eng.tAmb
  Constant8 : Constant  Value=genset.eng.fAmb
  Constant9 : Constant  Value=genset.eng.pBack
  Gain : Gain  Gain=genset.eng.omegaENom
  Gain1 : Gain  Gain=1/genset.eng.tqShaftNom
  InCylinderMV1 : Subsystem  mask{fs=genset.eng.fs, Vd=genset.eng.vD, LHV=genset.eng.LHV, Pe_nom=genset.eng.powNom, SFC=genset.eng.SFC, vol_eff_coeff1=genset.eng.volEff1, vol_eff_coeff2=genset.eng.volEff2, T_pe=genset.eng.tPe, nstroke=genset.eng.nStroke, m_f_cyc_max=genset.eng.mFCycMax, C1=genset.eng.C1, p_a_inf=genset.eng.pAInf, Pe0=genset.eng.powL0*genset.eng.powNom}
      mask prompts: fs "Stoichiometric fuel-air ratio"; Vd "Displacement volume (m3)"; LHV "Lower heating value of the fuel (J/kg)"; Pe_nom "Rated shaft power (W)"; SFC "Quadratic SFC curve coefficient (3x1)"; vol_eff_coeff1 "Volumetric efficiency coefficient for higher inlet pressure"; vol_eff_coeff2 "Volumetric efficiency coefficient for lower inlet pressure"; T_pe "Time constant for the torque development"; nstroke "Number of stroke"; m_f_cyc_max "Maximum amount of fuel injected per cycle (kg)"; C1 "Heat loss coefficient"; p_a_inf "Upper pressure limit for volumetric efficiency model 1 [bar]"; Pe0 "Initial power"
      mask TypeOptions fs: S-Function/fs
      mask TypeOptions Vd: S-Function/Vd
      mask TypeOptions LHV: S-Function/LHV
      mask TypeOptions Pe_nom: S-Function/Pe_nom
      mask TypeOptions SFC: S-Function/SFC
      mask TypeOptions vol_eff_coeff1: S-Function/vol_eff_coeff1
      mask TypeOptions vol_eff_coeff2: S-Function/vol_eff_coeff2
      mask TypeOptions T_pe: S-Function/T_pe
      mask TypeOptions nstroke: S-Function/nstroke
      mask TypeOptions m_f_cyc_max: S-Function/m_f_cyc_max
      mask TypeOptions C1: S-Function/C1
      mask TypeOptions p_a_inf: S-Function/p_a_inf
      mask TypeOptions Pe0: S-Function/Pe0
      mask Display: image(imread('figs/EngCyl.png'),'center')
  Sum{,1..8} (9 alike) : Sum  Inputs=-+|
  Terminator{,1..4} (5 alike) : Terminator
  TurbineMV1 : Subsystem  mask{fs=genset.eng.fs, flow_coeff_turb=genset.eng.flowCoeffTurb, D_turb_wheel=genset.eng.dTurbWheel, Uc_opt=genset.eng.ucOpt, eta_turb_max=genset.eng.effTurbMax, T_ref_turb=genset.eng.T_ref_turb}
      mask prompts: fs "Stoichiometric fuel-air ratio"; flow_coeff_turb "Flow coefficient for turbine model (3x1)"; D_turb_wheel "Turbine wheel diameter (m)"; Uc_opt "Optimal blade speed ratio"; eta_turb_max "Maximum efficiency"; T_ref_turb "Reference temperature"
      mask Display: image(imread('figs/turbine.png'),'center')
  TurbochargerShaft : Subsystem
  airReceiver : Subsystem  mask{fs=genset.eng.fs, m0=genset.eng.m0AR, E0=genset.eng.E0AR, mb0=genset.eng.mb0AR, V0=genset.eng.vAR}
      mask prompts: fs "Stoichiometric fuel-air ratio"; m0 "Initial mass (kg)"; E0 "Initial internal energy (J)"; mb0 "Initial burned fuel mass (kg)"; V0 "Initial volume (m3)"
      mask Display: image(imread('figs/Receiver.png'),'center')
  exhaustReceiver : Subsystem  mask{fs=genset.eng.fs, m0=genset.eng.m0ER, E0=genset.eng.E0ER, mb0=genset.eng.mb0ER, V0=genset.eng.vER}
      mask prompts: fs "Stoichiometric fuel-air ratio"; m0 "Initial mass (kg)"; E0 "Initial internal energy (J)"; mb0 "Initial burned fuel mass (kg)"; V0 "Initial volume (m3)"
      mask Display: image(imread('figs/Receiver.png'),'center')
  pipe : Subsystem  mask{fs=genset.eng.fs, m0=genset.eng.m0PipeAComp, E0=genset.eng.e0PipeAComp, mb0=genset.eng.mb0PipeAComp, V0=genset.eng.vPipeAComp}
      mask prompts: fs "Stoichiometric fuel-air ratio"; m0 "Initial mass (kg)"; E0 "Initial internal energy (J)"; mb0 "Initial burned fuel mass (kg)"; V0 "Initial volume (m3)"
      mask Display: image(imread('figs/pipe.png'),'center')
  Tqe : Outport
  powEffPu : Outport  Port=2
  volEff : Outport  Port=3
  pAR : Outport  Port=4
  TAR : Outport  Port=5
  wires:
  TurbineMV1/2(dmEmb_d) -> Terminator/1
  TurbineMV1/4(Td_calc) -> Terminator2/1
  TurbineMV1/5(eta_t) -> Terminator1/1
  Constant5/1 -> Bus Creator1/2, Bus Creator/2  "T"
  Constant8/1 -> Bus Creator1/3, Bus Creator/3  "F"
  Constant/1 -> Bus Creator/1  "p"
  Bus Creator1/1 -> [pTFATurb]
  Constant9/1 -> Bus Creator1/1  "p"
  Bus Selector3/2 -> Sum4/1  "<dEu>"
  [pTFBComp] -> CompressorNV/1(pTF_u)
  [pTFATurb] -> TurbineMV1/2(pTF_d)
  TurbineMV1/3(Tqt) -> [turbTq]
  Bus Selector3/3 -> Sum5/1  "<dmbu>"
  InCylinderMV1/1(dmEmbu) -> Bus Selector2/1
  Bus Selector2/1 -> Sum/1  "<dmu>"
  Sum/1 -> airReceiver/1(dm)  "dm"
  Bus Selector2/2 -> Sum1/1  "<dEu>"
  Bus Selector2/3 -> Sum2/1  "<dmbu>"
  exhaustReceiver/1(pTFV) -> InCylinderMV1/2(pTFd), TurbineMV1/1(pTF_u)
  omegaEngPu/1 -> Gain/1
  airReceiver/1(pTFV) -> InCylinderMV1/1(pTFu), Bus Selector/1, AirWaterCoolerNV/2(pTFd)
  Constant4/1 -> pipe/4(dV)
  Bus Selector1/2 -> Sum7/2  "<dEd>"
  Bus Selector1/3 -> Sum8/2  "<dmbd>"
  Bus Selector1/1 -> Sum6/2  "<dmd>"
  Bus Creator/1 -> [pTFBComp]
  Bus Selector3/1 -> Sum3/1  "<dmu>"
  [omegaT] -> TurbineMV1/3(omegat)
  TurbineMV1/1(dmEmb_u) -> Bus Selector3/1
  InCylinderMV1/5(pe_pu) -> powEffPu/1
  Sum6/1 -> pipe/1(dm)  "dm"
  AirWaterCoolerNV/2(dmEmbd) -> Bus Selector6/1
  Bus Selector8/2 -> Sum7/1  "<dEu>"
  Sum7/1 -> pipe/2(dE)
  Bus Selector8/1 -> Sum6/1  "<dmu>"
  Gain/1 -> InCylinderMV1/3(omegae)
  Sum8/1 -> pipe/3(dmb)
  pipe/1(pTFV) -> AirWaterCoolerNV/1(pTFu), CompressorNV/2(pTF_d)
  Bus Selector8/3 -> Sum8/1  "<dmbu>"
  AirWaterCoolerNV/1(dmEmbu) -> Bus Selector8/1
  Bus Selector6/1 -> Sum/2  "<dmd>"
  Bus Selector6/2 -> Sum1/2  "<dEd>"
  Sum3/1 -> exhaustReceiver/1(dm)  "dm"
  Constant2/1 -> exhaustReceiver/4(dV)
  Sum5/1 -> exhaustReceiver/3(dmb)
  Sum1/1 -> airReceiver/2(dE)
  Sum2/1 -> airReceiver/3(dmb)
  Bus Selector4/2 -> Sum4/2  "<dEd>"
  Sum4/1 -> exhaustReceiver/2(dE)
  InCylinderMV1/2(dmEmbd) -> Bus Selector4/1
  Bus Selector6/3 -> Sum2/2  "<dmbd>"
  Bus Selector4/3 -> Sum5/2  "<dmbd>"
  Constant1/1 -> airReceiver/4(dV)
  Bus Selector4/1 -> Sum3/2  "<dmd>"
  CompressorNV/2(dmEmb_d) -> Bus Selector1/1
  Constant3/1 -> AirWaterCoolerNV/3(TCW)
  InCylinderMV1/4(vol_eff) -> volEff/1
  uGov/1 -> InCylinderMV1/4(throttle)
  Gain1/1 -> Tqe/1
  Bus Selector/1 -> pAR/1  "<p>"
  Bus Selector/2 -> TAR/1  "<T>"
  CompressorNV/4(eta_c) -> Terminator3/1
  CompressorNV/1(dmEmb_u) -> Terminator4/1
  InCylinderMV1/3(Tqe) -> Gain1/1
  CompressorNV/3(Tqt) -> TurbochargerShaft/1(tqComp)  "tqComp"
  [turbTq] -> TurbochargerShaft/2(tqTurb)  "tqTurb"
  TurbochargerShaft/1(omegaTC) -> CompressorNV/3(omegat), [omegaT]  "omegaTC"

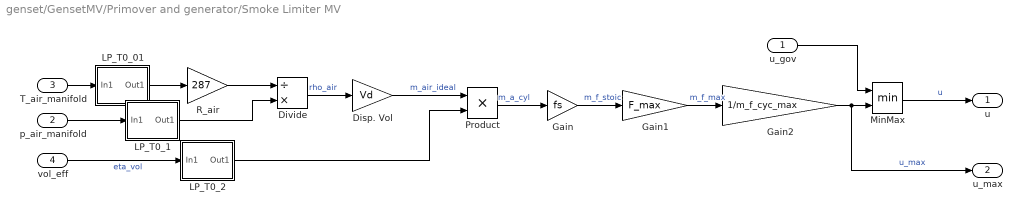
== system genset/GensetMV/Primover and generator/Smoke Limiter MV ==
  u_gov : Inport
  p_air_manifold : Inport  Port=2
  T_air_manifold : Inport  Port=3
  vol_eff : Inport  Port=4
  Disp. Vol : Gain  Gain=Vd
  Divide : Product  Inputs=/*
  Gain : Gain  Gain=fs
  Gain1 : Gain  Gain=F_max
  Gain2 : Gain  Gain=1/m_f_cyc_max
  LP_T0_01 : Subsystem
  LP_T0_1 : Subsystem
  LP_T0_2 : Subsystem
  MinMax : MinMax  Inputs=2
  Product : Product
  R_air : Gain  Gain=287
  u : Outport
  u_max : Outport  Port=2
  wires:
  LP_T0_2/1(Out1) -> Product/2
  LP_T0_1/1(Out1) -> Divide/2
  LP_T0_01/1(Out1) -> R_air/1
  Divide/1 -> Disp. Vol/1  "rho_air"
  p_air_manifold/1 -> LP_T0_1/1(In1)
  R_air/1 -> Divide/1
  T_air_manifold/1 -> LP_T0_01/1(In1)
  Disp. Vol/1 -> Product/1  "m_air_ideal"
  MinMax/1 -> u/1  "u"
  vol_eff/1 -> LP_T0_2/1(In1)  "eta_vol"
  Product/1 -> Gain/1  "m_a_cyl"
  u_gov/1 -> MinMax/1
  Gain/1 -> Gain1/1  "m_f_stoic"
  Gain1/1 -> Gain2/1  "m_f_max"
  Gain2/1 -> u_max/1, MinMax/2  "u_max"

== system genset/GensetMV/Primover and generator/Subsystem1 ==
  d/dt : Inport
  reset : Inport  Port=2
  x0 : Inport  Port=3
  Gain : Gain  Gain=1000
  Integrator : Integrator  InitialCondition=genset.theta0
  MATLAB Function : MATLAB Function  TreatAsAtomicUnit=on
  Sum : Sum  Inputs=-|+
  Switch : Switch  Threshold=1
  Out1 : Outport
  wires:
  Integrator/1 -> Out1/1, Sum/1
  reset/1 -> Switch/2
  x0/1 -> Sum/2
  Sum/1 -> MATLAB Function/1(u)
  Gain/1 -> Switch/3
  MATLAB Function/1(y) -> Gain/1
  d/dt/1 -> Switch/1
  Switch/1 -> Integrator/1

== system genset/Genset/Primover and generator/turbo/Derivative, low-passed ==
  u : Inport
  Gain : Gain  Gain=10
  Integrator : Integrator  InitialCondition=genset.u0
  Sum : Sum  Inputs=|+-
  du/dt : Outport
  wires:
  Sum/1 -> Gain/1
  Integrator/1 -> Sum/2
  Gain/1 -> du/dt/1, Integrator/1
  u/1 -> Sum/1

== system genset/Genset/Primover and generator/turbo/dead-band rate limiter ==
  u_d : Inport
  Constant : Constant  Value=umin
  Constant1 : Constant  Value=genset.governor.deltaU
  Delta : MATLAB Function  Commented=on  TreatAsAtomicUnit=on
  Gain : Gain  Gain=10
  Integrator : Integrator  InitialCondition=umax  LimitOutput=on  UpperSaturationLimit=umax  LowerSaturationLimit=umin
  Saturation : Saturate  UpperLimit=genset.governor.rampMax  LowerLimit=-.2
  Saturation Dynamic : simulink/Discontinuities/Saturation Dynamic  OutMin=[]  OutMax=[]  OutDataTypeStr=Inherit: Same as second input  OutDataType=fixdt(1, 16)  OutScaling=2^-10  DoSatur=off
  Sum : Sum  Inputs=|+++
  Sum1 : Sum  Inputs=-+|
  u_max : Outport
  u_saturated : Outport  Port=2
  wires:
  Gain/1 -> Saturation/1
  Sum1/1 -> Gain/1
  Sum/1 -> Sum1/2  "u+delta"
  Constant/1 -> Saturation Dynamic/3
  u_d/1 -> Saturation Dynamic/2  "ud"
  Integrator/1 -> u_max/1, Sum1/1, Saturation Dynamic/1  "umax"
  Saturation/1 -> Integrator/1
  Saturation Dynamic/1 -> Delta/1(p), Sum/1, u_saturated/1  "usat"
  Delta/1(delta) -> Sum/2
  Constant1/1 -> Sum/3

== system genset/GensetMV/Primover and generator/MVEM_TC/AirWaterCoolerNV ==
  pTFu : Inport
  pTFd : Inport  Port=2
  TCW : Inport  Port=3
  Bus Creator : BusCreator  Inputs=3
  Bus Creator1 : BusCreator  Inputs=3
  Bus Selector : BusSelector  OutputSignals=p,T,F
  Bus Selector1 : BusSelector  OutputSignals=p,T,F
  S-Function : S-Function  FunctionName=AirWaterCoolerPTF  Parameters=fs,Cd,A_air_path,dm_cw,coeff_T_cw_K,Cp_cw,D_cw_pipe  SFunctionModules='GetAirDensity GetAirThermalConduct GetAirViscosity GetCompCombGas_rtwutil GetHTCoeffHTX GetIdealNozzleFlow GetThdynCombGasZach rt_nonfinite rtGetInf rtGetNaN'  EnableBusSupport=off  mask{fs=fs, Cd=Cd, A_air_path=A_air_path, dm_cw=dm_cw, coeff_T_cw_K=coeff_T_cw_K, Cp_cw=Cp_cw, D_cw_pipe=D_cw_pipe}
      mask prompts: fs "Stoichiometric fuel-air ratio"; Cd "Discharge coefficient (0.8)"; A_air_path "Effective sectional area of air path (m2)"; dm_cw "Coolant flow rate (kg/s)"; coeff_T_cw_K "Coefficient for effective heat transfer area w.r.t. coolant temperature (2x1)"; Cp_cw "Specific heat capacity of coolant"; D_cw_pipe "Pipe diameter of the cooling water pipe in the cooler (m)"
  dmEmbu : Outport
  dmEmbd : Outport  Port=2
  wires:
  TCW/1 -> S-Function/7
  S-Function/1 -> Bus Creator/1  "dmu"
  S-Function/2 -> Bus Creator/2  "dEu"
  S-Function/3 -> Bus Creator/3  "dmbu"
  Bus Creator/1 -> dmEmbu/1
  S-Function/5 -> Bus Creator1/2  "dEd"
  S-Function/6 -> Bus Creator1/3  "dmbd"
  S-Function/4 -> Bus Creator1/1  "dmd"
  Bus Creator1/1 -> dmEmbd/1
  pTFu/1 -> Bus Selector/1
  pTFd/1 -> Bus Selector1/1
  Bus Selector/1 -> S-Function/1  "<p>"
  Bus Selector/2 -> S-Function/2  "<T>"
  Bus Selector/3 -> S-Function/3  "<F>"
  Bus Selector1/2 -> S-Function/5  "<T>"
  Bus Selector1/1 -> S-Function/4  "<p>"
  Bus Selector1/3 -> S-Function/6  "<F>"

== system genset/GensetMV/Primover and generator/MVEM_TC/CompressorNV ==
  pTF_u : Inport
  pTF_d : Inport  Port=2
  omegat : Inport  Port=3
  Bus Creator : BusCreator  Inputs=3
  Bus Creator1 : BusCreator  Inputs=3
  Bus Selector : BusSelector  OutputSignals=p,T,F
  Bus Selector1 : BusSelector  OutputSignals=p,T,F
  S-Function : S-Function  FunctionName=compressor_calc_PTF  Parameters=fs,comp_flow_map,comp_eff_map,pr_rep,n288_rep,int32(npr),int32(nsp)  SFunctionModules=GetThdynCombGasZach.c  EnableBusSupport=off
  dmEmb_u : Outport
  dmEmb_d : Outport  Port=2
  Tqt : Outport  Port=3
  eta_c : Outport  Port=4
  wires:
  pTF_d/1 -> Bus Selector1/1
  pTF_u/1 -> Bus Selector/1
  Bus Selector/2 -> S-Function/2  "<T>"
  Bus Selector/3 -> S-Function/3  "<F>"
  Bus Selector/1 -> S-Function/1  "<p>"
  Bus Selector1/2 -> S-Function/5  "<T>"
  Bus Selector1/3 -> S-Function/6  "<F>"
  Bus Selector1/1 -> S-Function/4  "<p>"
  omegat/1 -> S-Function/7
  S-Function/2 -> Bus Creator/2  "dEu"
  S-Function/1 -> Bus Creator/1  "dmu"
  S-Function/3 -> Bus Creator/3  "dmbu"
  S-Function/5 -> Bus Creator1/2  "dEd"
  S-Function/4 -> Bus Creator1/1  "dmd"
  S-Function/6 -> Bus Creator1/3  "dmbd"
  S-Function/7 -> Tqt/1
  S-Function/8 -> eta_c/1
  Bus Creator/1 -> dmEmb_u/1
  Bus Creator1/1 -> dmEmb_d/1

== system genset/GensetMV/Primover and generator/MVEM_TC/InCylinderMV1 ==
  pTFu : Inport
  pTFd : Inport  Port=2
  omegae : Inport  Port=3
  throttle : Inport  Port=4
  Bus Creator : BusCreator  Inputs=3
  Bus Creator1 : BusCreator  Inputs=3
  Bus Selector : BusSelector  OutputSignals=p,T,F
  Bus Selector1 : BusSelector  OutputSignals=p,T,F
  S-Function : S-Function  FunctionName=InCylinderMV  Parameters=fs,Vd,LHV,Pe_nom,SFC,vol_eff_coeff1,vol_eff_coeff2,T_pe,nstroke,m_f_cyc_max,C1,p_a_inf,Pe0  SFunctionModules='GetThdynCombGasZach'  EnableBusSupport=off  mask{fs=fs, Vd=Vd, LHV=LHV, Pe_nom=Pe_nom, SFC=SFC, vol_eff_coeff1=vol_eff_coeff1, vol_eff_coeff2=vol_eff_coeff2, T_pe=T_pe, nstroke=nstroke, m_f_cyc_max=m_f_cyc_max, C1=C1, p_a_inf=p_a_inf, Pe0=Pe0}
      mask prompts: fs "Stoichiometric fuel air ratio"; Vd "Displacement volume [m3]"; LHV "Low heating value of the fuel [J/kg]"; Pe_nom "Rated power [W]"; SFC "Coefficient for the SFC model"; vol_eff_coeff1 "Coefficient for volumetric efficiency model for higher pressure"; vol_eff_coeff2 "Coefficient for volumetric efficiency model for lower pressure"; T_pe "Time constant for power development (0.01)"; nstroke "Number of stroke"; m_f_cyc_max "Maximum injected fuel per cycle"; C1 "Cofficient of heat transfer"; p_a_inf "Upper pressure limit for vol. eff. model change"; Pe0 "Initial power load"
  dmEmbu : Outport
  dmEmbd : Outport  Port=2
  Tqe : Outport  Port=3
  vol_eff : Outport  Port=4
  pe_pu : Outport  Port=5
  wires:
  S-Function/8 -> vol_eff/1  "volEff"
  S-Function/7 -> Tqe/1
  Bus Creator1/1 -> dmEmbd/1
  Bus Creator/1 -> dmEmbu/1
  S-Function/3 -> Bus Creator/3  "dmbu"
  S-Function/2 -> Bus Creator/2  "dEu"
  S-Function/1 -> Bus Creator/1  "dmu"
  throttle/1 -> S-Function/8
  omegae/1 -> S-Function/7
  S-Function/9 -> pe_pu/1
  S-Function/4 -> Bus Creator1/1  "dmd"
  S-Function/6 -> Bus Creator1/3  "dmbd"
  S-Function/5 -> Bus Creator1/2  "dEd"
  pTFu/1 -> Bus Selector/1
  pTFd/1 -> Bus Selector1/1
  Bus Selector/2 -> S-Function/2  "<T>"
  Bus Selector/1 -> S-Function/1  "<p>"
  Bus Selector/3 -> S-Function/3  "<F>"
  Bus Selector1/2 -> S-Function/5  "<T>"
  Bus Selector1/1 -> S-Function/4  "<p>"
  Bus Selector1/3 -> S-Function/6  "<F>"

== system genset/GensetMV/Primover and generator/MVEM_TC/TurbineMV1 ==
  pTF_u : Inport
  pTF_d : Inport  Port=2
  omegat : Inport  Port=3
  Bus Creator : BusCreator  Inputs=3
  Bus Creator1 : BusCreator  Inputs=3
  Bus Selector : BusSelector  OutputSignals=p,T,F
  Bus Selector1 : BusSelector  OutputSignals=p,T,F
  S-Function : S-Function  FunctionName=turbine_calc_MV_PTF  Parameters=fs,flow_coeff_turb,D_turb_wheel,Uc_opt,eta_turb_max,T_ref_turb  SFunctionModules=GetThdynCombGasZach.c  EnableBusSupport=off
  dmEmb_u : Outport
  dmEmb_d : Outport  Port=2
  Tqt : Outport  Port=3
  Td_calc : Outport  Port=4
  eta_t : Outport  Port=5
  wires:
  pTF_u/1 -> Bus Selector/1
  Bus Selector/2 -> S-Function/2  "<T>"
  Bus Selector/3 -> S-Function/3  "<F>"
  Bus Selector/1 -> S-Function/1  "<p>"
  pTF_d/1 -> Bus Selector1/1
  Bus Selector1/2 -> S-Function/5  "<T>"
  Bus Selector1/3 -> S-Function/6  "<F>"
  Bus Selector1/1 -> S-Function/4  "<p>"
  omegat/1 -> S-Function/7
  S-Function/1 -> Bus Creator/1  "dmu"
  S-Function/2 -> Bus Creator/2  "dEu"
  S-Function/3 -> Bus Creator/3  "dmbu"
  Bus Creator/1 -> dmEmb_u/1
  S-Function/4 -> Bus Creator1/1  "dmd"
  S-Function/5 -> Bus Creator1/2  "dEd"
  S-Function/6 -> Bus Creator1/3  "dmbd"
  Bus Creator1/1 -> dmEmb_d/1
  S-Function/7 -> Tqt/1
  S-Function/8 -> Td_calc/1
  S-Function/9 -> eta_t/1

== system genset/GensetMV/Primover and generator/MVEM_TC/TurbochargerShaft ==
  tqComp : Inport
  tqTurb : Inport  Port=2
  Gain1 : Gain
  Gain3 : Gain  Gain=1/genset.eng.jTC
  Integrator : Integrator  InitialCondition=genset.eng.omegaT0*genset.eng.jTC
  Saturation : Saturate  UpperLimit=genset.eng.RPMtMax*pi/30*1.1;  LowerLimit=genset.eng.RPMtMax*pi/30*0.24;
  Sum10 : Sum  Inputs=-+|
  Sum9 : Sum  Inputs=-++
  omegaTC : Outport
  wires:
  tqComp/1 -> Sum9/1
  tqTurb/1 -> Sum9/2
  Sum9/1 -> Integrator/1
  Integrator/1 -> Gain3/1
  Gain3/1 -> Saturation/1, Sum10/1  "omegat"
  Sum10/1 -> Gain1/1
  Saturation/1 -> Sum10/2, omegaTC/1
  Gain1/1 -> Sum9/3

== system genset/GensetMV/Primover and generator/MVEM_TC/airReceiver ==
  dm : Inport
  dE : Inport  Port=2
  dmb : Inport  Port=3
  dV : Inport  Port=4
  Bus Creator : BusCreator
  S-Function : S-Function  FunctionName=ThdynCVNV  Parameters=fs,m0,E0,mb0,V0  SFunctionModules=GetThdynCombGasZach.c GetPTF.c  EnableBusSupport=off
  pTFV : Outport
  wires:
  dE/1 -> S-Function/2
  dm/1 -> S-Function/1
  dmb/1 -> S-Function/3
  dV/1 -> S-Function/4
  S-Function/2 -> Bus Creator/2  "T"
  S-Function/1 -> Bus Creator/1  "p"
  S-Function/3 -> Bus Creator/3  "F"
  S-Function/4 -> Bus Creator/4  "V"
  Bus Creator/1 -> pTFV/1
